simulink model "simulacion_control_trayectoria"  (R2023b)
settings: Solver=VariableStepAuto  StartTime=0.0  StopTime=25  MaxStep=0.001  RelTol=1e-3
undefined symbols (not defined in the file): X, Y, Z
libraries: sm_lib x85, nesl_utility x7
(part 3 of 3)

== matlab function simulacion_control_trayectoria/MATLAB Function1 ==
  data: t input; P output
function P = trayectoria(t)
% ==========================
% DEFINICIÓN DE WAYPOINTS
% ==========================
% wp = [
%     0    0    0.1
%     0    0    0.1
%     0    0    0.2
%     0.2  0    0.2
%     0.2  0.2  0.2
%    -0.2  0.2  0.2
%    -0.2 -0.2  0.2
%     0.2 -0.2  0.2
%     0.2  0    0.2
%     0    0    0.2
%     0    0    0.1
% ];

% S S I I
% I D I D

wp = [
    0    0    0   0
   0.8  0.8  0.8 0.8    % Levanta
  -3.3  3.3 -3.3 3.3    % Inclina en +X
   -1    7   -7  -1    % Inclina en +X +Y

   3.3   3.3   -3.3  -3.3    % Inclina en +Y
    7   -1   -1  -7    % Inclina en -X +Y

    3.3   -3.3    3.3  -3.3    % Inclina en -X
   -1   -7    7  -1    % Inclina en -X -Y

   -3.3   -3.3    3.3   3.3    % Inclina en -Y
   -7   -1   -1   7    % Inclina en +X -Y

   -3.3    3.3   -3.3   3.3    % Inclina en +X
   0.8  0.8  0.8 0.8    % Vuelve a altura levantada
];

% 0, 3, -3, 0 -> 0.05, 0.05, 0.111
% -1, 6, -6, 1 -> 0.118, 0.118, 0.121

% ==========================
% DURACIÓN POR TRAMO
% Debe haber N-1 tiempos
% ==========================
%Tseg = 5*[2 1 1 1 2 2 2 1 1 1];   % EJEMPLO → tú colocas lo que quieras
%Tseg = [5, 5, 5];   % EJEMPLO → tú colocas lo que quieras
Tseg = [2, 2, 2, 2, 2, 2, 2, 2, 2, 2, 2];


N = size(wp,1) - 1;           % Número de tramos

if length(Tseg) ~= N
    error('El vector Tseg debe tener %d elementos', N);
end

% ==========================
% TIEMPO ACUMULADO POR TRAMO
% ==========================
Tcum = [0, cumsum(Tseg)];

T_total = Tcum(end);

% ==========================
% CLAMP DE TIEMPO
% ==========================
if t <= 0
    P = wp(1,:);
    return;
elseif t >= T_total
    P = wp(end,:);
    return;
end

% ==========================
% DETERMINAR TRAMO ACTUAL
% ==========================
i = find(t >= Tcum(1:end-1) & t < Tcum(2:end), 1);

% Tiempo local del tramo
t0 = Tcum(i);
t1 = Tcum(i+1);
tau = (t - t0) / (t1 - t0);

% ==========================
% INTERPOLACIÓN LINEAL
% ==========================
p0 = wp(i,:);
p1 = wp(i+1,:);

p_int = p0 + tau * (p1 - p0);

P = [p_int(1), p_int(2), p_int(3), p_int(4)];
end

== matlab function simulacion_control_trayectoria/Efector Final/MATLAB Function1 ==
  data: R input; rpy output
function rpy = rot_to_rpy(R)
% INVERSA DE rpy_to_rot
% Convierte matriz de rotación (3x3) → roll, pitch, yaw (en grados)
% Convención: R = Rz(yaw) * Ry(pitch) * Rx(roll)

% --- Extraer elementos ---
r11 = R(1,1); r12 = R(1,2); r13 = R(1,3);
r21 = R(2,1); r22 = R(2,2); r23 = R(2,3);
r31 = R(3,1); r32 = R(3,2); r33 = R(3,3);

% --- Pitch ---
pitch = asin(-r31);

% Comprobar gimbal lock
if abs(cos(pitch)) > 1e-6
    roll  = atan2(r32, r33);
    yaw   = atan2(r21, r11);
else
    % Gimbal lock
    roll = 0;  % arbitrario
    if r31 == -1
        pitch =  pi/2;
        yaw = atan2(r12, r22);
    else
        pitch = -pi/2;
        yaw = atan2(-r12, -r22);
    end
end

% Convertir a grados
rpy = [roll pitch yaw] * 180/pi;
end
